simulink model "World_jessica_cs"  (R2019a)
settings: Solver=ode5  StartTime=0.0  StopTime=inf  FixedStep=1/60  RelTol=1e-3
PreLoadFcn:
  | mbxruntime.callbacks.PreLoadFcn(bdroot);
PostLoadFcn:
  | mbxruntime.callbacks.PostLoadFcn(bdroot);
InitFcn:
  | mbxruntime.callbacks.InitFcn(bdroot);
StartFcn:
  | mbxruntime.callbacks.StartFcn(bdroot);
StopFcn:
  | mbxruntime.callbacks.StopFcn(bdroot);
model workspace: external: MAT-File .\World_jessica_cs_hws.mat (data not in the file)
undefined symbols (not defined in the file or in its folder): DiscIntNeverNeededParam, InitImageOutputDir, mbxruntime, tabledata, World_jessica_cs_4acb408e0ac9f240, World_jessica_cs_800e508dbc53d9df, World_jessica_cs_Audi_A8_Sedan_1_Path_pathUniqueID, World_jessica_cs_bd1f9e0b3a3a0faa, World_jessica_cs_BMW_X5_SUV_1_Path_pathUniqueID, World_jessica_cs_BMW_X5_SUV_1_SpeedProfile_speedProfileUniqueID, World_jessica_cs_Boy_150_1_Path_pathUniqueID, World_jessica_cs_Boy_150_1_SpeedProfile_speedProfileUniqueID, World_jessica_cs_Citroen_C3_Hatchback_1_Path_pathUniqueID, World_jessica_cs_Male_CyclingCyclist_1_Path_pathUniqueID
libraries: adeye_lib x26, simulink_extras x24, simulink x2, PreScanUsefulBlocks x1
(part 4 of 7)

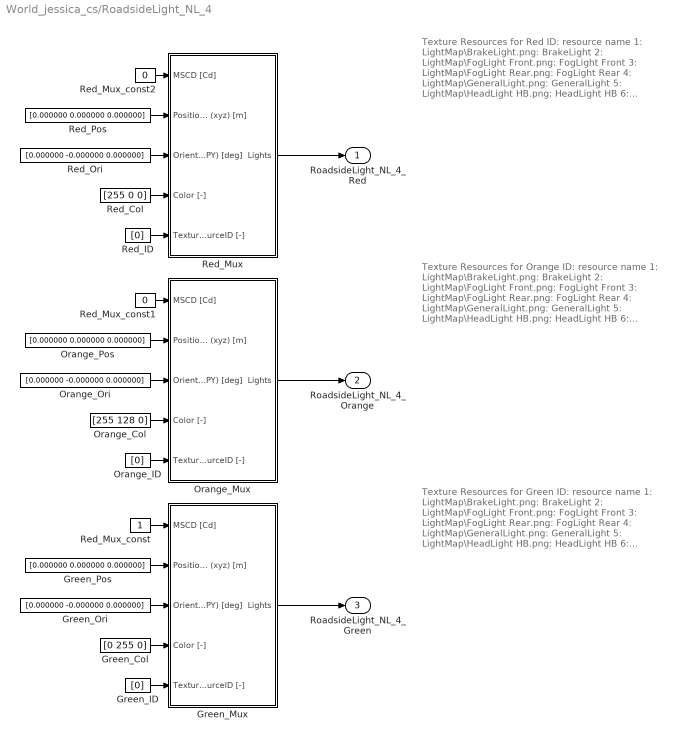
== system World_jessica_cs/RoadsideLight_NL_4 ==
  note: Texture Resources for Red
      |
      | ID: resource name
      | 1: LightMap\BrakeLight.png: BrakeLight
      | 2: LightMap\FogLight Front.png: FogLight Front
      | 3: LightMap\FogLight Rear.png: FogLight Rear
      | 4: LightMap\GeneralLight.png: GeneralLight
      | 5: LightMap\HeadLight HB.png: HeadLight HB
      | 6: LightMap\HeadLight LB.png: HeadLight LB
      | 7: LightMap\RearLight.png: RearLight
      | 8: LightMap\ReversingLight.png: ReversingLight
  note: Texture Resources for Orange
      |
      | ID: resource name
      | 1: LightMap\BrakeLight.png: BrakeLight
      | 2: LightMap\FogLight Front.png: FogLight Front
      | 3: LightMap\FogLight Rear.png: FogLight Rear
      | 4: LightMap\GeneralLight.png: GeneralLight
      | 5: LightMap\HeadLight HB.png: HeadLight HB
      | 6: LightMap\HeadLight LB.png: HeadLight LB
      | 7: LightMap\RearLight.png: RearLight
      | 8: LightMap\ReversingLight.png: ReversingLight
  note: Texture Resources for Green
      |
      | ID: resource name
      | 1: LightMap\BrakeLight.png: BrakeLight
      | 2: LightMap\FogLight Front.png: FogLight Front
      | 3: LightMap\FogLight Rear.png: FogLight Rear
      | 4: LightMap\GeneralLight.png: GeneralLight
      | 5: LightMap\HeadLight HB.png: HeadLight HB
      | 6: LightMap\HeadLight LB.png: HeadLight LB
      | 7: LightMap\RearLight.png: RearLight
      | 8: LightMap\ReversingLight.png: ReversingLight
  Green_Col : Constant  Tag=VisuLightConst  Value=[0 255 0]
  Green_ID : Constant  Tag=VisuLightConst  Value=[0]
  Green_Mux : Subsystem  Tag=mux/ActiveLight  mask(PreScan User Interface: VisuActiveLight){}
      mask help:
      | The VisuActiveLight block provides a way for detailed animation of Light Sources, such as the indicator, brake, fog and main lights of a vehicle, or a light post.
      |
      | For more information, please click Help.
      settings: DeleteFcn=PreScanBlockDeleteFcn;
      mask Help: eval('openHelp(209)')
  Green_Ori : Constant  Tag=VisuLightConst  Value=[0.000000 -0.000000 0.000000]
  Green_Pos : Constant  Tag=VisuLightConst  Value=[0.000000 0.000000 0.000000]
  Orange_Col : Constant  Tag=VisuLightConst  Value=[255 128 0]
  Orange_ID : Constant  Tag=VisuLightConst  Value=[0]
  Orange_Mux : Subsystem  Tag=mux/ActiveLight  mask(PreScan User Interface: VisuActiveLight){}
      mask help:
      | The VisuActiveLight block provides a way for detailed animation of Light Sources, such as the indicator, brake, fog and main lights of a vehicle, or a light post.
      |
      | For more information, please click Help.
      settings: DeleteFcn=PreScanBlockDeleteFcn;
      mask Help: eval('openHelp(209)')
  Orange_Ori : Constant  Tag=VisuLightConst  Value=[0.000000 -0.000000 0.000000]
  Orange_Pos : Constant  Tag=VisuLightConst  Value=[0.000000 0.000000 0.000000]
  Red_Col : Constant  Tag=VisuLightConst  Value=[255 0 0]
  Red_ID : Constant  Tag=VisuLightConst  Value=[0]
  Red_Mux : Subsystem  Tag=mux/ActiveLight  mask(PreScan User Interface: VisuActiveLight){}
      mask help:
      | The VisuActiveLight block provides a way for detailed animation of Light Sources, such as the indicator, brake, fog and main lights of a vehicle, or a light post.
      |
      | For more information, please click Help.
      settings: DeleteFcn=PreScanBlockDeleteFcn;
      mask Help: eval('openHelp(209)')
  Red_Mux_const : Constant  Tag=VisuLightConst
  Red_Mux_const1 : Constant  Tag=VisuLightConst  Value=0
  Red_Mux_const2 : Constant  Tag=VisuLightConst  Value=0
  Red_Ori : Constant  Tag=VisuLightConst  Value=[0.000000 -0.000000 0.000000]
  Red_Pos : Constant  Tag=VisuLightConst  Value=[0.000000 0.000000 0.000000]
  RoadsideLight_NL_4_Red : Outport  Tag=outport/Red  OutDataTypeStr=Bus: PRESCAN_VISULIGHTACTUATOR_DATA  SampleTime=1/60
  RoadsideLight_NL_4_Orange : Outport  Tag=outport/Orange  Port=2  OutDataTypeStr=Bus: PRESCAN_VISULIGHTACTUATOR_DATA  SampleTime=1/60
  RoadsideLight_NL_4_Green : Outport  Tag=outport/Green  Port=3  OutDataTypeStr=Bus: PRESCAN_VISULIGHTACTUATOR_DATA  SampleTime=1/60
  wires:
  Red_Mux_const2/1 -> Red_Mux/1(MSCD [Cd])
  Red_Mux_const1/1 -> Orange_Mux/1(MSCD [Cd])
  Red_Mux_const/1 -> Green_Mux/1(MSCD [Cd])
  Red_Mux/1(Lights) -> RoadsideLight_NL_4_Red/1
  Red_Pos/1 -> Red_Mux/2(Position (xyz) [m])
  Red_Ori/1 -> Red_Mux/3(Orientation (RPY) [deg])
  Red_Col/1 -> Red_Mux/4(Color [-])
  Red_ID/1 -> Red_Mux/5(TextureResourceID [-])
  Orange_Mux/1(Lights) -> RoadsideLight_NL_4_Orange/1
  Orange_Pos/1 -> Orange_Mux/2(Position (xyz) [m])
  Orange_Ori/1 -> Orange_Mux/3(Orientation (RPY) [deg])
  Orange_Col/1 -> Orange_Mux/4(Color [-])
  Orange_ID/1 -> Orange_Mux/5(TextureResourceID [-])
  Green_Mux/1(Lights) -> RoadsideLight_NL_4_Green/1
  Green_Pos/1 -> Green_Mux/2(Position (xyz) [m])
  Green_Ori/1 -> Green_Mux/3(Orientation (RPY) [deg])
  Green_Col/1 -> Green_Mux/4(Color [-])
  Green_ID/1 -> Green_Mux/5(TextureResourceID [-])

== system World_jessica_cs/RoadsideLight_NL_4_Green ==
  RoadsideLight_NL_4_Green : Inport  Tag=inport/Green  OutDataTypeStr=Bus: PRESCAN_VISULIGHTACTUATOR_DATA  SampleTime=1/60  BusOutputAsStruct=on
  Actuator : S-Function  FunctionName=sfun_VisuLightActuator  Parameters=mbxruntime.parameters.convert(UniqueID), mbxruntime.parameters.convert(LightName), mbxruntime.parameters.convert(PivotName), mbxruntime.parameters.convert(TextureResources), mbxruntime.parameters.convert(ColorsObjectName), mbxruntime.parameters.convert(MeshOnColor), mbxruntime.parameters.convert(MeshOffColor),tabledata, TimeStep  SFunctionDeploymentMode=off  EnableBusSupport=off  mask(PreScan Sink Block: VisuActiveLight){UniqueID=4878, LightName=RoadsideLight_NL_4.LightActuator_2_Green_ActiveLight, PivotName=RoadsideLight_NL_4.Green, TextureResources={ '1' 'LightMap\BrakeLight.png' '2' 'LightMap\FogLight Front.png' '3' 'LightMap\FogLight Rear.png' '4' 'LightMap\GeneralLight.png' '5' 'LightMap\HeadLight HB.png' '6' 'LightMap\HeadLight LB.png' '7' 'LightMap\RearLight.png' '8' 'LightMap\ReversingLight.png'}, ColorsObjectName=RoadsideLight_NL_4.Green, MeshOnColor=[0  100    0  255    0  100    0  255  102  102  102  255    0  510    0  255], MeshOffColor=[0  100    0  255    0  100    0  255  102  102  102  255    0    0    0  255], TimeStep=1/60}
      mask prompts: UniqueID "Parent Unique Identifier"; LightName "Light"; PivotName "Pivot"; TextureResources "Texture Resources"; ColorsObjectName "Light Fixture Color Object"; MeshOnColor "Light Fixture On Color"; MeshOffColor "Light Fixture Off Color"; TimeStep "Simulink time step"
      mask help:
      | The VisuActiveLight block provides a way for detailed animation of Light Sources, such as the indicator, brake, fog and main lights of a vehicle, or a light post.
      |
      | For more information, please click Help.
      mask init:
      | [tabledata] = mbxruntime.parameters.table(UniqueID,LightName,PivotName,TextureResources,ColorsObjectName,MeshOnColor,MeshOffColor);
      mask Help: eval('openHelp(209)')
      mask Display: image(imread('HeadLight.png'))
  wires:
  RoadsideLight_NL_4_Green/1 -> Actuator/1

== system World_jessica_cs/RoadsideLight_NL_4_Orange ==
  RoadsideLight_NL_4_Orange : Inport  Tag=inport/Orange  OutDataTypeStr=Bus: PRESCAN_VISULIGHTACTUATOR_DATA  SampleTime=1/60  BusOutputAsStruct=on
  Actuator : S-Function  FunctionName=sfun_VisuLightActuator  Parameters=mbxruntime.parameters.convert(UniqueID), mbxruntime.parameters.convert(LightName), mbxruntime.parameters.convert(PivotName), mbxruntime.parameters.convert(TextureResources), mbxruntime.parameters.convert(ColorsObjectName), mbxruntime.parameters.convert(MeshOnColor), mbxruntime.parameters.convert(MeshOffColor),tabledata, TimeStep  SFunctionDeploymentMode=off  EnableBusSupport=off  mask(PreScan Sink Block: VisuActiveLight){UniqueID=4878, LightName=RoadsideLight_NL_4.LightActuator_1_Orange_ActiveLight, PivotName=RoadsideLight_NL_4.Orange, TextureResources={ '1' 'LightMap\BrakeLight.png' '2' 'LightMap\FogLight Front.png' '3' 'LightMap\FogLight Rear.png' '4' 'LightMap\GeneralLight.png' '5' 'LightMap\HeadLight HB.png' '6' 'LightMap\HeadLight LB.png' '7' 'LightMap\RearLight.png' '8' 'LightMap\ReversingLight.png'}, ColorsObjectName=RoadsideLight_NL_4.Orange, MeshOnColor=[100   50    0  255  100   50    0  255  102  102  102  255  510  256    0  255], MeshOffColor=[100   50    0  255  100   50    0  255  102  102  102  255    0    0    0  255], TimeStep=1/60}
      mask prompts: UniqueID "Parent Unique Identifier"; LightName "Light"; PivotName "Pivot"; TextureResources "Texture Resources"; ColorsObjectName "Light Fixture Color Object"; MeshOnColor "Light Fixture On Color"; MeshOffColor "Light Fixture Off Color"; TimeStep "Simulink time step"
      mask help:
      | The VisuActiveLight block provides a way for detailed animation of Light Sources, such as the indicator, brake, fog and main lights of a vehicle, or a light post.
      |
      | For more information, please click Help.
      mask init:
      | [tabledata] = mbxruntime.parameters.table(UniqueID,LightName,PivotName,TextureResources,ColorsObjectName,MeshOnColor,MeshOffColor);
      mask Help: eval('openHelp(209)')
      mask Display: image(imread('HeadLight.png'))
  wires:
  RoadsideLight_NL_4_Orange/1 -> Actuator/1

== system World_jessica_cs/RoadsideLight_NL_4_Red ==
  RoadsideLight_NL_4_Red : Inport  Tag=inport/Red  OutDataTypeStr=Bus: PRESCAN_VISULIGHTACTUATOR_DATA  SampleTime=1/60  BusOutputAsStruct=on
  Actuator : S-Function  FunctionName=sfun_VisuLightActuator  Parameters=mbxruntime.parameters.convert(UniqueID), mbxruntime.parameters.convert(LightName), mbxruntime.parameters.convert(PivotName), mbxruntime.parameters.convert(TextureResources), mbxruntime.parameters.convert(ColorsObjectName), mbxruntime.parameters.convert(MeshOnColor), mbxruntime.parameters.convert(MeshOffColor),tabledata, TimeStep  SFunctionDeploymentMode=off  EnableBusSupport=off  mask(PreScan Sink Block: VisuActiveLight){UniqueID=4878, LightName=RoadsideLight_NL_4.LightActuator_0_Red_ActiveLight, PivotName=RoadsideLight_NL_4.Red, TextureResources={ '1' 'LightMap\BrakeLight.png' '2' 'LightMap\FogLight Front.png' '3' 'LightMap\FogLight Rear.png' '4' 'LightMap\GeneralLight.png' '5' 'LightMap\HeadLight HB.png' '6' 'LightMap\HeadLight LB.png' '7' 'LightMap\RearLight.png' '8' 'LightMap\ReversingLight.png'}, ColorsObjectName=RoadsideLight_NL_4.Red, MeshOnColor=[100    0    0  255  100    0    0  255  102  102  102  255  510    0    0  255], MeshOffColor=[100    0    0  255  100    0    0  255  102  102  102  255    0    0    0  255], TimeStep=1/60}
      mask prompts: UniqueID "Parent Unique Identifier"; LightName "Light"; PivotName "Pivot"; TextureResources "Texture Resources"; ColorsObjectName "Light Fixture Color Object"; MeshOnColor "Light Fixture On Color"; MeshOffColor "Light Fixture Off Color"; TimeStep "Simulink time step"
      mask help:
      | The VisuActiveLight block provides a way for detailed animation of Light Sources, such as the indicator, brake, fog and main lights of a vehicle, or a light post.
      |
      | For more information, please click Help.
      mask init:
      | [tabledata] = mbxruntime.parameters.table(UniqueID,LightName,PivotName,TextureResources,ColorsObjectName,MeshOnColor,MeshOffColor);
      mask Help: eval('openHelp(209)')
      mask Display: image(imread('HeadLight.png'))
  wires:
  RoadsideLight_NL_4_Red/1 -> Actuator/1

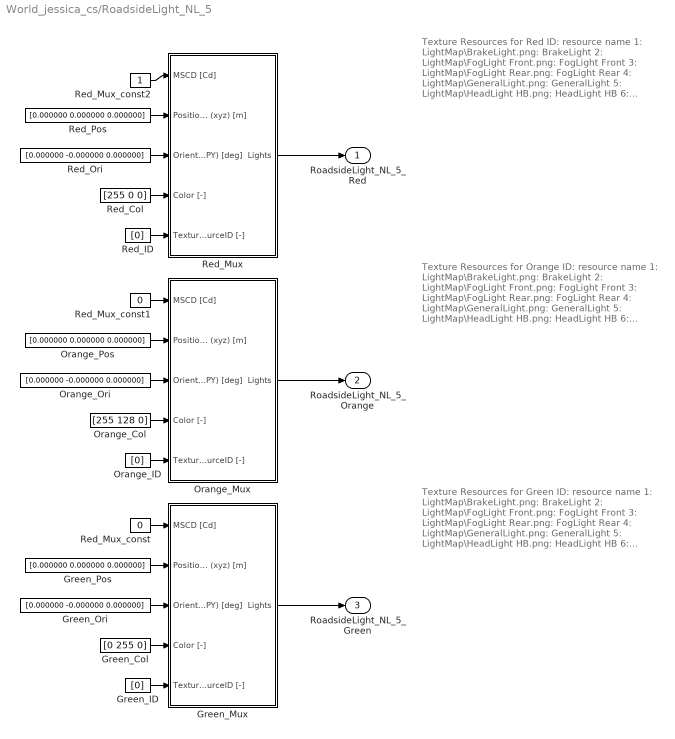
== system World_jessica_cs/RoadsideLight_NL_5 ==
  note: Texture Resources for Red
      |
      | ID: resource name
      | 1: LightMap\BrakeLight.png: BrakeLight
      | 2: LightMap\FogLight Front.png: FogLight Front
      | 3: LightMap\FogLight Rear.png: FogLight Rear
      | 4: LightMap\GeneralLight.png: GeneralLight
      | 5: LightMap\HeadLight HB.png: HeadLight HB
      | 6: LightMap\HeadLight LB.png: HeadLight LB
      | 7: LightMap\RearLight.png: RearLight
      | 8: LightMap\ReversingLight.png: ReversingLight
  note: Texture Resources for Orange
      |
      | ID: resource name
      | 1: LightMap\BrakeLight.png: BrakeLight
      | 2: LightMap\FogLight Front.png: FogLight Front
      | 3: LightMap\FogLight Rear.png: FogLight Rear
      | 4: LightMap\GeneralLight.png: GeneralLight
      | 5: LightMap\HeadLight HB.png: HeadLight HB
      | 6: LightMap\HeadLight LB.png: HeadLight LB
      | 7: LightMap\RearLight.png: RearLight
      | 8: LightMap\ReversingLight.png: ReversingLight
  note: Texture Resources for Green
      |
      | ID: resource name
      | 1: LightMap\BrakeLight.png: BrakeLight
      | 2: LightMap\FogLight Front.png: FogLight Front
      | 3: LightMap\FogLight Rear.png: FogLight Rear
      | 4: LightMap\GeneralLight.png: GeneralLight
      | 5: LightMap\HeadLight HB.png: HeadLight HB
      | 6: LightMap\HeadLight LB.png: HeadLight LB
      | 7: LightMap\RearLight.png: RearLight
      | 8: LightMap\ReversingLight.png: ReversingLight
  Green_Col : Constant  Tag=VisuLightConst  Value=[0 255 0]
  Green_ID : Constant  Tag=VisuLightConst  Value=[0]
  Green_Mux : Subsystem  Tag=mux/ActiveLight  mask(PreScan User Interface: VisuActiveLight){}
      mask help:
      | The VisuActiveLight block provides a way for detailed animation of Light Sources, such as the indicator, brake, fog and main lights of a vehicle, or a light post.
      |
      | For more information, please click Help.
      settings: DeleteFcn=PreScanBlockDeleteFcn;
      mask Help: eval('openHelp(209)')
  Green_Ori : Constant  Tag=VisuLightConst  Value=[0.000000 -0.000000 0.000000]
  Green_Pos : Constant  Tag=VisuLightConst  Value=[0.000000 0.000000 0.000000]
  Orange_Col : Constant  Tag=VisuLightConst  Value=[255 128 0]
  Orange_ID : Constant  Tag=VisuLightConst  Value=[0]
  Orange_Mux : Subsystem  Tag=mux/ActiveLight  mask(PreScan User Interface: VisuActiveLight){}
      mask help:
      | The VisuActiveLight block provides a way for detailed animation of Light Sources, such as the indicator, brake, fog and main lights of a vehicle, or a light post.
      |
      | For more information, please click Help.
      settings: DeleteFcn=PreScanBlockDeleteFcn;
      mask Help: eval('openHelp(209)')
  Orange_Ori : Constant  Tag=VisuLightConst  Value=[0.000000 -0.000000 0.000000]
  Orange_Pos : Constant  Tag=VisuLightConst  Value=[0.000000 0.000000 0.000000]
  Red_Col : Constant  Tag=VisuLightConst  Value=[255 0 0]
  Red_ID : Constant  Tag=VisuLightConst  Value=[0]
  Red_Mux : Subsystem  Tag=mux/ActiveLight  mask(PreScan User Interface: VisuActiveLight){}
      mask help:
      | The VisuActiveLight block provides a way for detailed animation of Light Sources, such as the indicator, brake, fog and main lights of a vehicle, or a light post.
      |
      | For more information, please click Help.
      settings: DeleteFcn=PreScanBlockDeleteFcn;
      mask Help: eval('openHelp(209)')
  Red_Mux_const : Constant  Tag=VisuLightConst  Value=0
  Red_Mux_const1 : Constant  Tag=VisuLightConst  Value=0
  Red_Mux_const2 : Constant  Tag=VisuLightConst
  Red_Ori : Constant  Tag=VisuLightConst  Value=[0.000000 -0.000000 0.000000]
  Red_Pos : Constant  Tag=VisuLightConst  Value=[0.000000 0.000000 0.000000]
  RoadsideLight_NL_5_Red : Outport  Tag=outport/Red  OutDataTypeStr=Bus: PRESCAN_VISULIGHTACTUATOR_DATA  SampleTime=1/60
  RoadsideLight_NL_5_Orange : Outport  Tag=outport/Orange  Port=2  OutDataTypeStr=Bus: PRESCAN_VISULIGHTACTUATOR_DATA  SampleTime=1/60
  RoadsideLight_NL_5_Green : Outport  Tag=outport/Green  Port=3  OutDataTypeStr=Bus: PRESCAN_VISULIGHTACTUATOR_DATA  SampleTime=1/60
  wires:
  Red_Mux_const2/1 -> Red_Mux/1(MSCD [Cd])
  Red_Mux_const1/1 -> Orange_Mux/1(MSCD [Cd])
  Red_Mux_const/1 -> Green_Mux/1(MSCD [Cd])
  Red_Mux/1(Lights) -> RoadsideLight_NL_5_Red/1
  Red_Pos/1 -> Red_Mux/2(Position (xyz) [m])
  Red_Ori/1 -> Red_Mux/3(Orientation (RPY) [deg])
  Red_Col/1 -> Red_Mux/4(Color [-])
  Red_ID/1 -> Red_Mux/5(TextureResourceID [-])
  Orange_Mux/1(Lights) -> RoadsideLight_NL_5_Orange/1
  Orange_Pos/1 -> Orange_Mux/2(Position (xyz) [m])
  Orange_Ori/1 -> Orange_Mux/3(Orientation (RPY) [deg])
  Orange_Col/1 -> Orange_Mux/4(Color [-])
  Orange_ID/1 -> Orange_Mux/5(TextureResourceID [-])
  Green_Mux/1(Lights) -> RoadsideLight_NL_5_Green/1
  Green_Pos/1 -> Green_Mux/2(Position (xyz) [m])
  Green_Ori/1 -> Green_Mux/3(Orientation (RPY) [deg])
  Green_Col/1 -> Green_Mux/4(Color [-])
  Green_ID/1 -> Green_Mux/5(TextureResourceID [-])

== system World_jessica_cs/RoadsideLight_NL_5_Green ==
  RoadsideLight_NL_5_Green : Inport  Tag=inport/Green  OutDataTypeStr=Bus: PRESCAN_VISULIGHTACTUATOR_DATA  SampleTime=1/60  BusOutputAsStruct=on
  Actuator : S-Function  FunctionName=sfun_VisuLightActuator  Parameters=mbxruntime.parameters.convert(UniqueID), mbxruntime.parameters.convert(LightName), mbxruntime.parameters.convert(PivotName), mbxruntime.parameters.convert(TextureResources), mbxruntime.parameters.convert(ColorsObjectName), mbxruntime.parameters.convert(MeshOnColor), mbxruntime.parameters.convert(MeshOffColor),tabledata, TimeStep  SFunctionDeploymentMode=off  EnableBusSupport=off  mask(PreScan Sink Block: VisuActiveLight){UniqueID=4879, LightName=RoadsideLight_NL_5.LightActuator_2_Green_ActiveLight, PivotName=RoadsideLight_NL_5.Green, TextureResources={ '1' 'LightMap\BrakeLight.png' '2' 'LightMap\FogLight Front.png' '3' 'LightMap\FogLight Rear.png' '4' 'LightMap\GeneralLight.png' '5' 'LightMap\HeadLight HB.png' '6' 'LightMap\HeadLight LB.png' '7' 'LightMap\RearLight.png' '8' 'LightMap\ReversingLight.png'}, ColorsObjectName=RoadsideLight_NL_5.Green, MeshOnColor=[0  100    0  255    0  100    0  255  102  102  102  255    0  510    0  255], MeshOffColor=[0  100    0  255    0  100    0  255  102  102  102  255    0    0    0  255], TimeStep=1/60}
      mask prompts: UniqueID "Parent Unique Identifier"; LightName "Light"; PivotName "Pivot"; TextureResources "Texture Resources"; ColorsObjectName "Light Fixture Color Object"; MeshOnColor "Light Fixture On Color"; MeshOffColor "Light Fixture Off Color"; TimeStep "Simulink time step"
      mask help:
      | The VisuActiveLight block provides a way for detailed animation of Light Sources, such as the indicator, brake, fog and main lights of a vehicle, or a light post.
      |
      | For more information, please click Help.
      mask init:
      | [tabledata] = mbxruntime.parameters.table(UniqueID,LightName,PivotName,TextureResources,ColorsObjectName,MeshOnColor,MeshOffColor);
      mask Help: eval('openHelp(209)')
      mask Display: image(imread('HeadLight.png'))
  wires:
  RoadsideLight_NL_5_Green/1 -> Actuator/1

== system World_jessica_cs/RoadsideLight_NL_5_Orange ==
  RoadsideLight_NL_5_Orange : Inport  Tag=inport/Orange  OutDataTypeStr=Bus: PRESCAN_VISULIGHTACTUATOR_DATA  SampleTime=1/60  BusOutputAsStruct=on
  Actuator : S-Function  FunctionName=sfun_VisuLightActuator  Parameters=mbxruntime.parameters.convert(UniqueID), mbxruntime.parameters.convert(LightName), mbxruntime.parameters.convert(PivotName), mbxruntime.parameters.convert(TextureResources), mbxruntime.parameters.convert(ColorsObjectName), mbxruntime.parameters.convert(MeshOnColor), mbxruntime.parameters.convert(MeshOffColor),tabledata, TimeStep  SFunctionDeploymentMode=off  EnableBusSupport=off  mask(PreScan Sink Block: VisuActiveLight){UniqueID=4879, LightName=RoadsideLight_NL_5.LightActuator_1_Orange_ActiveLight, PivotName=RoadsideLight_NL_5.Orange, TextureResources={ '1' 'LightMap\BrakeLight.png' '2' 'LightMap\FogLight Front.png' '3' 'LightMap\FogLight Rear.png' '4' 'LightMap\GeneralLight.png' '5' 'LightMap\HeadLight HB.png' '6' 'LightMap\HeadLight LB.png' '7' 'LightMap\RearLight.png' '8' 'LightMap\ReversingLight.png'}, ColorsObjectName=RoadsideLight_NL_5.Orange, MeshOnColor=[100   50    0  255  100   50    0  255  102  102  102  255  510  256    0  255], MeshOffColor=[100   50    0  255  100   50    0  255  102  102  102  255    0    0    0  255], TimeStep=1/60}
      mask prompts: UniqueID "Parent Unique Identifier"; LightName "Light"; PivotName "Pivot"; TextureResources "Texture Resources"; ColorsObjectName "Light Fixture Color Object"; MeshOnColor "Light Fixture On Color"; MeshOffColor "Light Fixture Off Color"; TimeStep "Simulink time step"
      mask help:
      | The VisuActiveLight block provides a way for detailed animation of Light Sources, such as the indicator, brake, fog and main lights of a vehicle, or a light post.
      |
      | For more information, please click Help.
      mask init:
      | [tabledata] = mbxruntime.parameters.table(UniqueID,LightName,PivotName,TextureResources,ColorsObjectName,MeshOnColor,MeshOffColor);
      mask Help: eval('openHelp(209)')
      mask Display: image(imread('HeadLight.png'))
  wires:
  RoadsideLight_NL_5_Orange/1 -> Actuator/1

== system World_jessica_cs/RoadsideLight_NL_5_Red ==
  RoadsideLight_NL_5_Red : Inport  Tag=inport/Red  OutDataTypeStr=Bus: PRESCAN_VISULIGHTACTUATOR_DATA  SampleTime=1/60  BusOutputAsStruct=on
  Actuator : S-Function  FunctionName=sfun_VisuLightActuator  Parameters=mbxruntime.parameters.convert(UniqueID), mbxruntime.parameters.convert(LightName), mbxruntime.parameters.convert(PivotName), mbxruntime.parameters.convert(TextureResources), mbxruntime.parameters.convert(ColorsObjectName), mbxruntime.parameters.convert(MeshOnColor), mbxruntime.parameters.convert(MeshOffColor),tabledata, TimeStep  SFunctionDeploymentMode=off  EnableBusSupport=off  mask(PreScan Sink Block: VisuActiveLight){UniqueID=4879, LightName=RoadsideLight_NL_5.LightActuator_0_Red_ActiveLight, PivotName=RoadsideLight_NL_5.Red, TextureResources={ '1' 'LightMap\BrakeLight.png' '2' 'LightMap\FogLight Front.png' '3' 'LightMap\FogLight Rear.png' '4' 'LightMap\GeneralLight.png' '5' 'LightMap\HeadLight HB.png' '6' 'LightMap\HeadLight LB.png' '7' 'LightMap\RearLight.png' '8' 'LightMap\ReversingLight.png'}, ColorsObjectName=RoadsideLight_NL_5.Red, MeshOnColor=[100    0    0  255  100    0    0  255  102  102  102  255  510    0    0  255], MeshOffColor=[100    0    0  255  100    0    0  255  102  102  102  255    0    0    0  255], TimeStep=1/60}
      mask prompts: UniqueID "Parent Unique Identifier"; LightName "Light"; PivotName "Pivot"; TextureResources "Texture Resources"; ColorsObjectName "Light Fixture Color Object"; MeshOnColor "Light Fixture On Color"; MeshOffColor "Light Fixture Off Color"; TimeStep "Simulink time step"
      mask help:
      | The VisuActiveLight block provides a way for detailed animation of Light Sources, such as the indicator, brake, fog and main lights of a vehicle, or a light post.
      |
      | For more information, please click Help.
      mask init:
      | [tabledata] = mbxruntime.parameters.table(UniqueID,LightName,PivotName,TextureResources,ColorsObjectName,MeshOnColor,MeshOffColor);
      mask Help: eval('openHelp(209)')
      mask Display: image(imread('HeadLight.png'))
  wires:
  RoadsideLight_NL_5_Red/1 -> Actuator/1

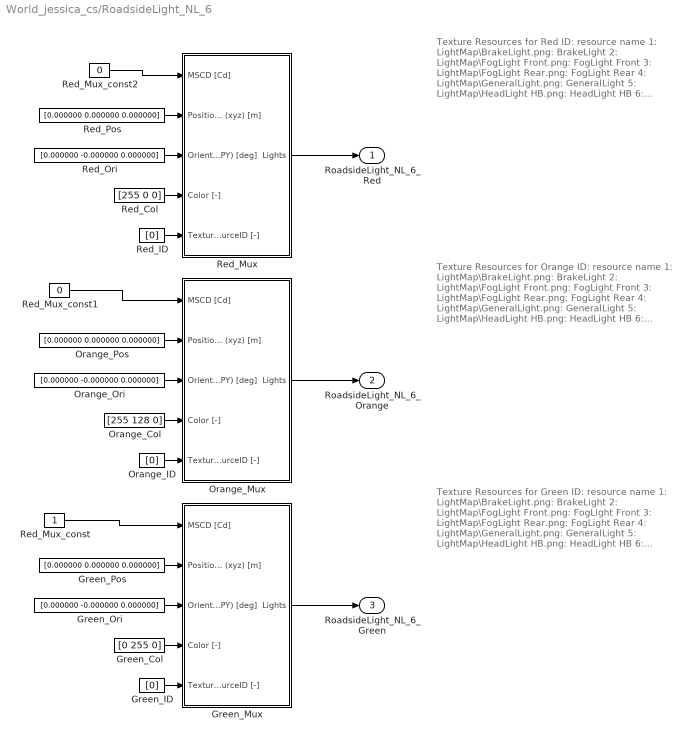
== system World_jessica_cs/RoadsideLight_NL_6 ==
  note: Texture Resources for Red
      |
      | ID: resource name
      | 1: LightMap\BrakeLight.png: BrakeLight
      | 2: LightMap\FogLight Front.png: FogLight Front
      | 3: LightMap\FogLight Rear.png: FogLight Rear
      | 4: LightMap\GeneralLight.png: GeneralLight
      | 5: LightMap\HeadLight HB.png: HeadLight HB
      | 6: LightMap\HeadLight LB.png: HeadLight LB
      | 7: LightMap\RearLight.png: RearLight
      | 8: LightMap\ReversingLight.png: ReversingLight
  note: Texture Resources for Orange
      |
      | ID: resource name
      | 1: LightMap\BrakeLight.png: BrakeLight
      | 2: LightMap\FogLight Front.png: FogLight Front
      | 3: LightMap\FogLight Rear.png: FogLight Rear
      | 4: LightMap\GeneralLight.png: GeneralLight
      | 5: LightMap\HeadLight HB.png: HeadLight HB
      | 6: LightMap\HeadLight LB.png: HeadLight LB
      | 7: LightMap\RearLight.png: RearLight
      | 8: LightMap\ReversingLight.png: ReversingLight
  note: Texture Resources for Green
      |
      | ID: resource name
      | 1: LightMap\BrakeLight.png: BrakeLight
      | 2: LightMap\FogLight Front.png: FogLight Front
      | 3: LightMap\FogLight Rear.png: FogLight Rear
      | 4: LightMap\GeneralLight.png: GeneralLight
      | 5: LightMap\HeadLight HB.png: HeadLight HB
      | 6: LightMap\HeadLight LB.png: HeadLight LB
      | 7: LightMap\RearLight.png: RearLight
      | 8: LightMap\ReversingLight.png: ReversingLight
  Green_Col : Constant  Tag=VisuLightConst  Value=[0 255 0]
  Green_ID : Constant  Tag=VisuLightConst  Value=[0]
  Green_Mux : Subsystem  Tag=mux/ActiveLight  mask(PreScan User Interface: VisuActiveLight){}
      mask help:
      | The VisuActiveLight block provides a way for detailed animation of Light Sources, such as the indicator, brake, fog and main lights of a vehicle, or a light post.
      |
      | For more information, please click Help.
      settings: DeleteFcn=PreScanBlockDeleteFcn;
      mask Help: eval('openHelp(209)')
  Green_Ori : Constant  Tag=VisuLightConst  Value=[0.000000 -0.000000 0.000000]
  Green_Pos : Constant  Tag=VisuLightConst  Value=[0.000000 0.000000 0.000000]
  Orange_Col : Constant  Tag=VisuLightConst  Value=[255 128 0]
  Orange_ID : Constant  Tag=VisuLightConst  Value=[0]
  Orange_Mux : Subsystem  Tag=mux/ActiveLight  mask(PreScan User Interface: VisuActiveLight){}
      mask help:
      | The VisuActiveLight block provides a way for detailed animation of Light Sources, such as the indicator, brake, fog and main lights of a vehicle, or a light post.
      |
      | For more information, please click Help.
      settings: DeleteFcn=PreScanBlockDeleteFcn;
      mask Help: eval('openHelp(209)')
  Orange_Ori : Constant  Tag=VisuLightConst  Value=[0.000000 -0.000000 0.000000]
  Orange_Pos : Constant  Tag=VisuLightConst  Value=[0.000000 0.000000 0.000000]
  Red_Col : Constant  Tag=VisuLightConst  Value=[255 0 0]
  Red_ID : Constant  Tag=VisuLightConst  Value=[0]
  Red_Mux : Subsystem  Tag=mux/ActiveLight  mask(PreScan User Interface: VisuActiveLight){}
      mask help:
      | The VisuActiveLight block provides a way for detailed animation of Light Sources, such as the indicator, brake, fog and main lights of a vehicle, or a light post.
      |
      | For more information, please click Help.
      settings: DeleteFcn=PreScanBlockDeleteFcn;
      mask Help: eval('openHelp(209)')
  Red_Mux_const : Constant  Tag=VisuLightConst
  Red_Mux_const1 : Constant  Tag=VisuLightConst  Value=0
  Red_Mux_const2 : Constant  Tag=VisuLightConst  Value=0
  Red_Ori : Constant  Tag=VisuLightConst  Value=[0.000000 -0.000000 0.000000]
  Red_Pos : Constant  Tag=VisuLightConst  Value=[0.000000 0.000000 0.000000]
  RoadsideLight_NL_6_Red : Outport  Tag=outport/Red  OutDataTypeStr=Bus: PRESCAN_VISULIGHTACTUATOR_DATA  SampleTime=1/60
  RoadsideLight_NL_6_Orange : Outport  Tag=outport/Orange  Port=2  OutDataTypeStr=Bus: PRESCAN_VISULIGHTACTUATOR_DATA  SampleTime=1/60
  RoadsideLight_NL_6_Green : Outport  Tag=outport/Green  Port=3  OutDataTypeStr=Bus: PRESCAN_VISULIGHTACTUATOR_DATA  SampleTime=1/60
  wires:
  Red_Mux_const2/1 -> Red_Mux/1(MSCD [Cd])
  Red_Mux_const1/1 -> Orange_Mux/1(MSCD [Cd])
  Red_Mux_const/1 -> Green_Mux/1(MSCD [Cd])
  Red_Mux/1(Lights) -> RoadsideLight_NL_6_Red/1
  Red_Pos/1 -> Red_Mux/2(Position (xyz) [m])
  Red_Ori/1 -> Red_Mux/3(Orientation (RPY) [deg])
  Red_Col/1 -> Red_Mux/4(Color [-])
  Red_ID/1 -> Red_Mux/5(TextureResourceID [-])
  Orange_Mux/1(Lights) -> RoadsideLight_NL_6_Orange/1
  Orange_Pos/1 -> Orange_Mux/2(Position (xyz) [m])
  Orange_Ori/1 -> Orange_Mux/3(Orientation (RPY) [deg])
  Orange_Col/1 -> Orange_Mux/4(Color [-])
  Orange_ID/1 -> Orange_Mux/5(TextureResourceID [-])
  Green_Mux/1(Lights) -> RoadsideLight_NL_6_Green/1
  Green_Pos/1 -> Green_Mux/2(Position (xyz) [m])
  Green_Ori/1 -> Green_Mux/3(Orientation (RPY) [deg])
  Green_Col/1 -> Green_Mux/4(Color [-])
  Green_ID/1 -> Green_Mux/5(TextureResourceID [-])

== system World_jessica_cs/RoadsideLight_NL_6_Green ==
  RoadsideLight_NL_6_Green : Inport  Tag=inport/Green  OutDataTypeStr=Bus: PRESCAN_VISULIGHTACTUATOR_DATA  SampleTime=1/60  BusOutputAsStruct=on
  Actuator : S-Function  FunctionName=sfun_VisuLightActuator  Parameters=mbxruntime.parameters.convert(UniqueID), mbxruntime.parameters.convert(LightName), mbxruntime.parameters.convert(PivotName), mbxruntime.parameters.convert(TextureResources), mbxruntime.parameters.convert(ColorsObjectName), mbxruntime.parameters.convert(MeshOnColor), mbxruntime.parameters.convert(MeshOffColor),tabledata, TimeStep  SFunctionDeploymentMode=off  EnableBusSupport=off  mask(PreScan Sink Block: VisuActiveLight){UniqueID=4880, LightName=RoadsideLight_NL_6.LightActuator_2_Green_ActiveLight, PivotName=RoadsideLight_NL_6.Green, TextureResources={ '1' 'LightMap\BrakeLight.png' '2' 'LightMap\FogLight Front.png' '3' 'LightMap\FogLight Rear.png' '4' 'LightMap\GeneralLight.png' '5' 'LightMap\HeadLight HB.png' '6' 'LightMap\HeadLight LB.png' '7' 'LightMap\RearLight.png' '8' 'LightMap\ReversingLight.png'}, ColorsObjectName=RoadsideLight_NL_6.Green, MeshOnColor=[0  100    0  255    0  100    0  255  102  102  102  255    0  510    0  255], MeshOffColor=[0  100    0  255    0  100    0  255  102  102  102  255    0    0    0  255], TimeStep=1/60}
      mask prompts: UniqueID "Parent Unique Identifier"; LightName "Light"; PivotName "Pivot"; TextureResources "Texture Resources"; ColorsObjectName "Light Fixture Color Object"; MeshOnColor "Light Fixture On Color"; MeshOffColor "Light Fixture Off Color"; TimeStep "Simulink time step"
      mask help:
      | The VisuActiveLight block provides a way for detailed animation of Light Sources, such as the indicator, brake, fog and main lights of a vehicle, or a light post.
      |
      | For more information, please click Help.
      mask init:
      | [tabledata] = mbxruntime.parameters.table(UniqueID,LightName,PivotName,TextureResources,ColorsObjectName,MeshOnColor,MeshOffColor);
      mask Help: eval('openHelp(209)')
      mask Display: image(imread('HeadLight.png'))
  wires:
  RoadsideLight_NL_6_Green/1 -> Actuator/1

== system World_jessica_cs/RoadsideLight_NL_6_Orange ==
  RoadsideLight_NL_6_Orange : Inport  Tag=inport/Orange  OutDataTypeStr=Bus: PRESCAN_VISULIGHTACTUATOR_DATA  SampleTime=1/60  BusOutputAsStruct=on
  Actuator : S-Function  FunctionName=sfun_VisuLightActuator  Parameters=mbxruntime.parameters.convert(UniqueID), mbxruntime.parameters.convert(LightName), mbxruntime.parameters.convert(PivotName), mbxruntime.parameters.convert(TextureResources), mbxruntime.parameters.convert(ColorsObjectName), mbxruntime.parameters.convert(MeshOnColor), mbxruntime.parameters.convert(MeshOffColor),tabledata, TimeStep  SFunctionDeploymentMode=off  EnableBusSupport=off  mask(PreScan Sink Block: VisuActiveLight){UniqueID=4880, LightName=RoadsideLight_NL_6.LightActuator_1_Orange_ActiveLight, PivotName=RoadsideLight_NL_6.Orange, TextureResources={ '1' 'LightMap\BrakeLight.png' '2' 'LightMap\FogLight Front.png' '3' 'LightMap\FogLight Rear.png' '4' 'LightMap\GeneralLight.png' '5' 'LightMap\HeadLight HB.png' '6' 'LightMap\HeadLight LB.png' '7' 'LightMap\RearLight.png' '8' 'LightMap\ReversingLight.png'}, ColorsObjectName=RoadsideLight_NL_6.Orange, MeshOnColor=[100   50    0  255  100   50    0  255  102  102  102  255  510  256    0  255], MeshOffColor=[100   50    0  255  100   50    0  255  102  102  102  255    0    0    0  255], TimeStep=1/60}
      mask prompts: UniqueID "Parent Unique Identifier"; LightName "Light"; PivotName "Pivot"; TextureResources "Texture Resources"; ColorsObjectName "Light Fixture Color Object"; MeshOnColor "Light Fixture On Color"; MeshOffColor "Light Fixture Off Color"; TimeStep "Simulink time step"
      mask help:
      | The VisuActiveLight block provides a way for detailed animation of Light Sources, such as the indicator, brake, fog and main lights of a vehicle, or a light post.
      |
      | For more information, please click Help.
      mask init:
      | [tabledata] = mbxruntime.parameters.table(UniqueID,LightName,PivotName,TextureResources,ColorsObjectName,MeshOnColor,MeshOffColor);
      mask Help: eval('openHelp(209)')
      mask Display: image(imread('HeadLight.png'))
  wires:
  RoadsideLight_NL_6_Orange/1 -> Actuator/1

== system World_jessica_cs/RoadsideLight_NL_6_Red ==
  RoadsideLight_NL_6_Red : Inport  Tag=inport/Red  OutDataTypeStr=Bus: PRESCAN_VISULIGHTACTUATOR_DATA  SampleTime=1/60  BusOutputAsStruct=on
  Actuator : S-Function  FunctionName=sfun_VisuLightActuator  Parameters=mbxruntime.parameters.convert(UniqueID), mbxruntime.parameters.convert(LightName), mbxruntime.parameters.convert(PivotName), mbxruntime.parameters.convert(TextureResources), mbxruntime.parameters.convert(ColorsObjectName), mbxruntime.parameters.convert(MeshOnColor), mbxruntime.parameters.convert(MeshOffColor),tabledata, TimeStep  SFunctionDeploymentMode=off  EnableBusSupport=off  mask(PreScan Sink Block: VisuActiveLight){UniqueID=4880, LightName=RoadsideLight_NL_6.LightActuator_0_Red_ActiveLight, PivotName=RoadsideLight_NL_6.Red, TextureResources={ '1' 'LightMap\BrakeLight.png' '2' 'LightMap\FogLight Front.png' '3' 'LightMap\FogLight Rear.png' '4' 'LightMap\GeneralLight.png' '5' 'LightMap\HeadLight HB.png' '6' 'LightMap\HeadLight LB.png' '7' 'LightMap\RearLight.png' '8' 'LightMap\ReversingLight.png'}, ColorsObjectName=RoadsideLight_NL_6.Red, MeshOnColor=[100    0    0  255  100    0    0  255  102  102  102  255  510    0    0  255], MeshOffColor=[100    0    0  255  100    0    0  255  102  102  102  255    0    0    0  255], TimeStep=1/60}
      mask prompts: UniqueID "Parent Unique Identifier"; LightName "Light"; PivotName "Pivot"; TextureResources "Texture Resources"; ColorsObjectName "Light Fixture Color Object"; MeshOnColor "Light Fixture On Color"; MeshOffColor "Light Fixture Off Color"; TimeStep "Simulink time step"
      mask help:
      | The VisuActiveLight block provides a way for detailed animation of Light Sources, such as the indicator, brake, fog and main lights of a vehicle, or a light post.
      |
      | For more information, please click Help.
      mask init:
      | [tabledata] = mbxruntime.parameters.table(UniqueID,LightName,PivotName,TextureResources,ColorsObjectName,MeshOnColor,MeshOffColor);
      mask Help: eval('openHelp(209)')
      mask Display: image(imread('HeadLight.png'))
  wires:
  RoadsideLight_NL_6_Red/1 -> Actuator/1

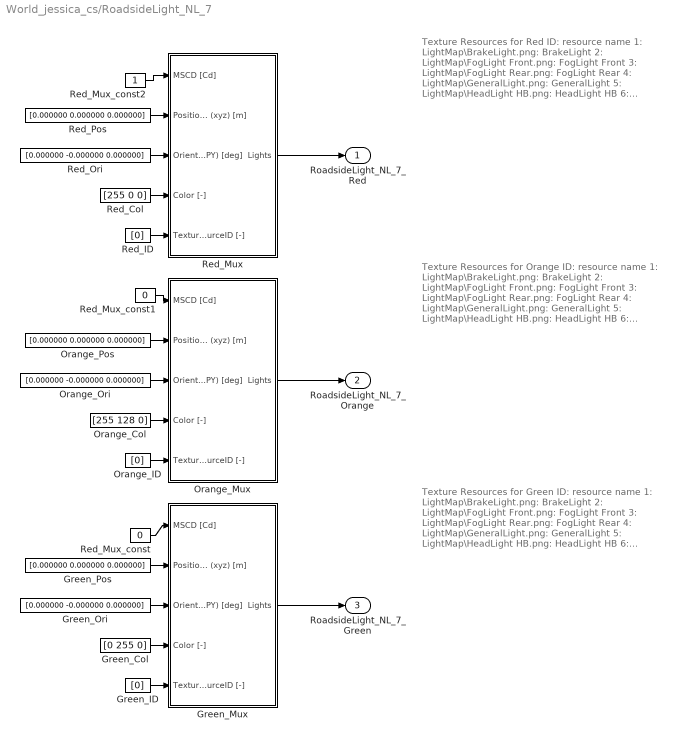
== system World_jessica_cs/RoadsideLight_NL_7 ==
  note: Texture Resources for Red
      |
      | ID: resource name
      | 1: LightMap\BrakeLight.png: BrakeLight
      | 2: LightMap\FogLight Front.png: FogLight Front
      | 3: LightMap\FogLight Rear.png: FogLight Rear
      | 4: LightMap\GeneralLight.png: GeneralLight
      | 5: LightMap\HeadLight HB.png: HeadLight HB
      | 6: LightMap\HeadLight LB.png: HeadLight LB
      | 7: LightMap\RearLight.png: RearLight
      | 8: LightMap\ReversingLight.png: ReversingLight
  note: Texture Resources for Orange
      |
      | ID: resource name
      | 1: LightMap\BrakeLight.png: BrakeLight
      | 2: LightMap\FogLight Front.png: FogLight Front
      | 3: LightMap\FogLight Rear.png: FogLight Rear
      | 4: LightMap\GeneralLight.png: GeneralLight
      | 5: LightMap\HeadLight HB.png: HeadLight HB
      | 6: LightMap\HeadLight LB.png: HeadLight LB
      | 7: LightMap\RearLight.png: RearLight
      | 8: LightMap\ReversingLight.png: ReversingLight
  note: Texture Resources for Green
      |
      | ID: resource name
      | 1: LightMap\BrakeLight.png: BrakeLight
      | 2: LightMap\FogLight Front.png: FogLight Front
      | 3: LightMap\FogLight Rear.png: FogLight Rear
      | 4: LightMap\GeneralLight.png: GeneralLight
      | 5: LightMap\HeadLight HB.png: HeadLight HB
      | 6: LightMap\HeadLight LB.png: HeadLight LB
      | 7: LightMap\RearLight.png: RearLight
      | 8: LightMap\ReversingLight.png: ReversingLight
  Green_Col : Constant  Tag=VisuLightConst  Value=[0 255 0]
  Green_ID : Constant  Tag=VisuLightConst  Value=[0]
  Green_Mux : Subsystem  Tag=mux/ActiveLight  mask(PreScan User Interface: VisuActiveLight){}
      mask help:
      | The VisuActiveLight block provides a way for detailed animation of Light Sources, such as the indicator, brake, fog and main lights of a vehicle, or a light post.
      |
      | For more information, please click Help.
      settings: DeleteFcn=PreScanBlockDeleteFcn;
      mask Help: eval('openHelp(209)')
  Green_Ori : Constant  Tag=VisuLightConst  Value=[0.000000 -0.000000 0.000000]
  Green_Pos : Constant  Tag=VisuLightConst  Value=[0.000000 0.000000 0.000000]
  Orange_Col : Constant  Tag=VisuLightConst  Value=[255 128 0]
  Orange_ID : Constant  Tag=VisuLightConst  Value=[0]
  Orange_Mux : Subsystem  Tag=mux/ActiveLight  mask(PreScan User Interface: VisuActiveLight){}
      mask help:
      | The VisuActiveLight block provides a way for detailed animation of Light Sources, such as the indicator, brake, fog and main lights of a vehicle, or a light post.
      |
      | For more information, please click Help.
      settings: DeleteFcn=PreScanBlockDeleteFcn;
      mask Help: eval('openHelp(209)')
  Orange_Ori : Constant  Tag=VisuLightConst  Value=[0.000000 -0.000000 0.000000]
  Orange_Pos : Constant  Tag=VisuLightConst  Value=[0.000000 0.000000 0.000000]
  Red_Col : Constant  Tag=VisuLightConst  Value=[255 0 0]
  Red_ID : Constant  Tag=VisuLightConst  Value=[0]
  Red_Mux : Subsystem  Tag=mux/ActiveLight  mask(PreScan User Interface: VisuActiveLight){}
      mask help:
      | The VisuActiveLight block provides a way for detailed animation of Light Sources, such as the indicator, brake, fog and main lights of a vehicle, or a light post.
      |
      | For more information, please click Help.
      settings: DeleteFcn=PreScanBlockDeleteFcn;
      mask Help: eval('openHelp(209)')
  Red_Mux_const : Constant  Tag=VisuLightConst  Value=0
  Red_Mux_const1 : Constant  Tag=VisuLightConst  Value=0
  Red_Mux_const2 : Constant  Tag=VisuLightConst
  Red_Ori : Constant  Tag=VisuLightConst  Value=[0.000000 -0.000000 0.000000]
  Red_Pos : Constant  Tag=VisuLightConst  Value=[0.000000 0.000000 0.000000]
  RoadsideLight_NL_7_Red : Outport  Tag=outport/Red  OutDataTypeStr=Bus: PRESCAN_VISULIGHTACTUATOR_DATA  SampleTime=1/60
  RoadsideLight_NL_7_Orange : Outport  Tag=outport/Orange  Port=2  OutDataTypeStr=Bus: PRESCAN_VISULIGHTACTUATOR_DATA  SampleTime=1/60
  RoadsideLight_NL_7_Green : Outport  Tag=outport/Green  Port=3  OutDataTypeStr=Bus: PRESCAN_VISULIGHTACTUATOR_DATA  SampleTime=1/60
  wires:
  Red_Mux_const2/1 -> Red_Mux/1(MSCD [Cd])
  Red_Mux_const1/1 -> Orange_Mux/1(MSCD [Cd])
  Red_Mux_const/1 -> Green_Mux/1(MSCD [Cd])
  Red_Mux/1(Lights) -> RoadsideLight_NL_7_Red/1
  Red_Pos/1 -> Red_Mux/2(Position (xyz) [m])
  Red_Ori/1 -> Red_Mux/3(Orientation (RPY) [deg])
  Red_Col/1 -> Red_Mux/4(Color [-])
  Red_ID/1 -> Red_Mux/5(TextureResourceID [-])
  Orange_Mux/1(Lights) -> RoadsideLight_NL_7_Orange/1
  Orange_Pos/1 -> Orange_Mux/2(Position (xyz) [m])
  Orange_Ori/1 -> Orange_Mux/3(Orientation (RPY) [deg])
  Orange_Col/1 -> Orange_Mux/4(Color [-])
  Orange_ID/1 -> Orange_Mux/5(TextureResourceID [-])
  Green_Mux/1(Lights) -> RoadsideLight_NL_7_Green/1
  Green_Pos/1 -> Green_Mux/2(Position (xyz) [m])
  Green_Ori/1 -> Green_Mux/3(Orientation (RPY) [deg])
  Green_Col/1 -> Green_Mux/4(Color [-])
  Green_ID/1 -> Green_Mux/5(TextureResourceID [-])

== system World_jessica_cs/RoadsideLight_NL_7_Green ==
  RoadsideLight_NL_7_Green : Inport  Tag=inport/Green  OutDataTypeStr=Bus: PRESCAN_VISULIGHTACTUATOR_DATA  SampleTime=1/60  BusOutputAsStruct=on
  Actuator : S-Function  FunctionName=sfun_VisuLightActuator  Parameters=mbxruntime.parameters.convert(UniqueID), mbxruntime.parameters.convert(LightName), mbxruntime.parameters.convert(PivotName), mbxruntime.parameters.convert(TextureResources), mbxruntime.parameters.convert(ColorsObjectName), mbxruntime.parameters.convert(MeshOnColor), mbxruntime.parameters.convert(MeshOffColor),tabledata, TimeStep  SFunctionDeploymentMode=off  EnableBusSupport=off  mask(PreScan Sink Block: VisuActiveLight){UniqueID=4881, LightName=RoadsideLight_NL_7.LightActuator_2_Green_ActiveLight, PivotName=RoadsideLight_NL_7.Green, TextureResources={ '1' 'LightMap\BrakeLight.png' '2' 'LightMap\FogLight Front.png' '3' 'LightMap\FogLight Rear.png' '4' 'LightMap\GeneralLight.png' '5' 'LightMap\HeadLight HB.png' '6' 'LightMap\HeadLight LB.png' '7' 'LightMap\RearLight.png' '8' 'LightMap\ReversingLight.png'}, ColorsObjectName=RoadsideLight_NL_7.Green, MeshOnColor=[0  100    0  255    0  100    0  255  102  102  102  255    0  510    0  255], MeshOffColor=[0  100    0  255    0  100    0  255  102  102  102  255    0    0    0  255], TimeStep=1/60}
      mask prompts: UniqueID "Parent Unique Identifier"; LightName "Light"; PivotName "Pivot"; TextureResources "Texture Resources"; ColorsObjectName "Light Fixture Color Object"; MeshOnColor "Light Fixture On Color"; MeshOffColor "Light Fixture Off Color"; TimeStep "Simulink time step"
      mask help:
      | The VisuActiveLight block provides a way for detailed animation of Light Sources, such as the indicator, brake, fog and main lights of a vehicle, or a light post.
      |
      | For more information, please click Help.
      mask init:
      | [tabledata] = mbxruntime.parameters.table(UniqueID,LightName,PivotName,TextureResources,ColorsObjectName,MeshOnColor,MeshOffColor);
      mask Help: eval('openHelp(209)')
      mask Display: image(imread('HeadLight.png'))
  wires:
  RoadsideLight_NL_7_Green/1 -> Actuator/1

== system World_jessica_cs/RoadsideLight_NL_7_Orange ==
  RoadsideLight_NL_7_Orange : Inport  Tag=inport/Orange  OutDataTypeStr=Bus: PRESCAN_VISULIGHTACTUATOR_DATA  SampleTime=1/60  BusOutputAsStruct=on
  Actuator : S-Function  FunctionName=sfun_VisuLightActuator  Parameters=mbxruntime.parameters.convert(UniqueID), mbxruntime.parameters.convert(LightName), mbxruntime.parameters.convert(PivotName), mbxruntime.parameters.convert(TextureResources), mbxruntime.parameters.convert(ColorsObjectName), mbxruntime.parameters.convert(MeshOnColor), mbxruntime.parameters.convert(MeshOffColor),tabledata, TimeStep  SFunctionDeploymentMode=off  EnableBusSupport=off  mask(PreScan Sink Block: VisuActiveLight){UniqueID=4881, LightName=RoadsideLight_NL_7.LightActuator_1_Orange_ActiveLight, PivotName=RoadsideLight_NL_7.Orange, TextureResources={ '1' 'LightMap\BrakeLight.png' '2' 'LightMap\FogLight Front.png' '3' 'LightMap\FogLight Rear.png' '4' 'LightMap\GeneralLight.png' '5' 'LightMap\HeadLight HB.png' '6' 'LightMap\HeadLight LB.png' '7' 'LightMap\RearLight.png' '8' 'LightMap\ReversingLight.png'}, ColorsObjectName=RoadsideLight_NL_7.Orange, MeshOnColor=[100   50    0  255  100   50    0  255  102  102  102  255  510  256    0  255], MeshOffColor=[100   50    0  255  100   50    0  255  102  102  102  255    0    0    0  255], TimeStep=1/60}
      mask prompts: UniqueID "Parent Unique Identifier"; LightName "Light"; PivotName "Pivot"; TextureResources "Texture Resources"; ColorsObjectName "Light Fixture Color Object"; MeshOnColor "Light Fixture On Color"; MeshOffColor "Light Fixture Off Color"; TimeStep "Simulink time step"
      mask help:
      | The VisuActiveLight block provides a way for detailed animation of Light Sources, such as the indicator, brake, fog and main lights of a vehicle, or a light post.
      |
      | For more information, please click Help.
      mask init:
      | [tabledata] = mbxruntime.parameters.table(UniqueID,LightName,PivotName,TextureResources,ColorsObjectName,MeshOnColor,MeshOffColor);
      mask Help: eval('openHelp(209)')
      mask Display: image(imread('HeadLight.png'))
  wires:
  RoadsideLight_NL_7_Orange/1 -> Actuator/1

== system World_jessica_cs/RoadsideLight_NL_7_Red ==
  RoadsideLight_NL_7_Red : Inport  Tag=inport/Red  OutDataTypeStr=Bus: PRESCAN_VISULIGHTACTUATOR_DATA  SampleTime=1/60  BusOutputAsStruct=on
  Actuator : S-Function  FunctionName=sfun_VisuLightActuator  Parameters=mbxruntime.parameters.convert(UniqueID), mbxruntime.parameters.convert(LightName), mbxruntime.parameters.convert(PivotName), mbxruntime.parameters.convert(TextureResources), mbxruntime.parameters.convert(ColorsObjectName), mbxruntime.parameters.convert(MeshOnColor), mbxruntime.parameters.convert(MeshOffColor),tabledata, TimeStep  SFunctionDeploymentMode=off  EnableBusSupport=off  mask(PreScan Sink Block: VisuActiveLight){UniqueID=4881, LightName=RoadsideLight_NL_7.LightActuator_0_Red_ActiveLight, PivotName=RoadsideLight_NL_7.Red, TextureResources={ '1' 'LightMap\BrakeLight.png' '2' 'LightMap\FogLight Front.png' '3' 'LightMap\FogLight Rear.png' '4' 'LightMap\GeneralLight.png' '5' 'LightMap\HeadLight HB.png' '6' 'LightMap\HeadLight LB.png' '7' 'LightMap\RearLight.png' '8' 'LightMap\ReversingLight.png'}, ColorsObjectName=RoadsideLight_NL_7.Red, MeshOnColor=[100    0    0  255  100    0    0  255  102  102  102  255  510    0    0  255], MeshOffColor=[100    0    0  255  100    0    0  255  102  102  102  255    0    0    0  255], TimeStep=1/60}
      mask prompts: UniqueID "Parent Unique Identifier"; LightName "Light"; PivotName "Pivot"; TextureResources "Texture Resources"; ColorsObjectName "Light Fixture Color Object"; MeshOnColor "Light Fixture On Color"; MeshOffColor "Light Fixture Off Color"; TimeStep "Simulink time step"
      mask help:
      | The VisuActiveLight block provides a way for detailed animation of Light Sources, such as the indicator, brake, fog and main lights of a vehicle, or a light post.
      |
      | For more information, please click Help.
      mask init:
      | [tabledata] = mbxruntime.parameters.table(UniqueID,LightName,PivotName,TextureResources,ColorsObjectName,MeshOnColor,MeshOffColor);
      mask Help: eval('openHelp(209)')
      mask Display: image(imread('HeadLight.png'))
  wires:
  RoadsideLight_NL_7_Red/1 -> Actuator/1
